simulink model "VentilatorClosedLoop_gas_f"  (R2018b)
settings: Solver=ode23t  StartTime=0.0  StopTime=50  MaxStep=0.001  RelTol=1e-3  EnableMultiTasking=on
PreLoadFcn:
  | loadVars
values from neighbouring files (symbols this model uses):
  basePSI = 14.7    [loadVars.m]
  D = 0.001    [loadVars.m]
  I = 0.2    [loadVars.m]
  P = 0.2    [loadVars.m]
libraries: fl_lib x26, nesl_utility x9, simulink x2, dspstat3 x1
(part 1 of 3)
settings Model: Creator=szhang  LastModifiedBy=etzorako
settings OptimizationCC: UseDivisionForNetSlopeComputation=on  LifeSpan=inf
settings DebuggingCC: LibraryContextMissingDiagnostic=none  SFUnexpectedBacktrackingDiag=warning  SFNoUnconditionalDefaultTransitionDiag=warning  SFExecutionAtInitializationDiag=none
settings SFSimCC: SimUseLocalCustomCode=off
settings RTWCC: RTWUseLocalCustomCode=off
settings CodeAppCC: StateflowObjectComments=on
settings GRTTargetCC: TargetLangStandard=C89/C90 (ANSI)  GeneratePreprocessorConditionals=Disable all
settings ConfigComp: CovMetricSettings=dw  CovHtmlReporting=on  CovSaveCumulativeToWorkspaceVar=on  CovSaveSingleToWorkspaceVar=on  CovExternalEMLEnable=off
settings SimscapeCC: SimscapeNormalizeSystem=off  SimscapeLogLimitData=off

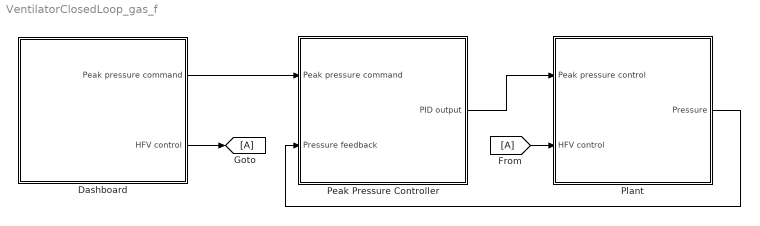
== system VentilatorClosedLoop_gas_f ==
  Dashboard : Subsystem
  Peak Pressure Controller : Subsystem
  Plant : Subsystem
  wires:
  [A] -> Plant/2(HFV control)
  Plant/1(Pressure) -> Peak Pressure Controller/2(Pressure feedback)
  Peak Pressure Controller/1(PID output) -> Plant/1(Peak pressure control)
  Dashboard/1(Peak pressure command) -> Peak Pressure Controller/1(Peak pressure command)
  Dashboard/2(HFV control) -> [A]

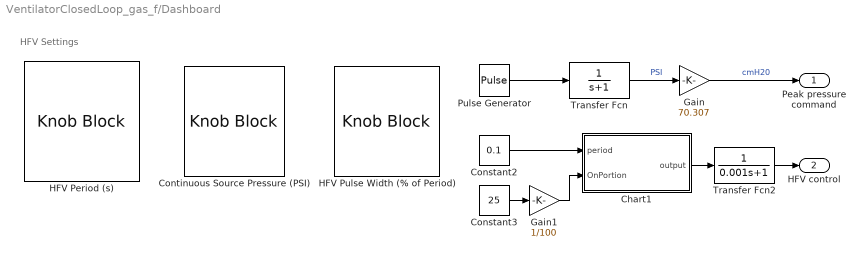
== system VentilatorClosedLoop_gas_f/Dashboard ==
  note: HFV Settings
  Chart1 : Stateflow chart  TreatAsAtomicUnit=on
  Constant2 : Constant  Value=0.1
  Constant3 : Constant  Value=25
  Continuous Source Pressure (PSI) : KnobBlock  WebBlockId=345  LabelPosition=Hide  ScaleMax=70  TickInterval=5
  Gain : Gain  Gain=70.307
  Gain1 : Gain  Gain=1/100
  HFV Period (s) : KnobBlock  WebBlockId=340  LabelPosition=Hide  ScaleMin=0.050000000000000003  ScaleMax=1  TickInterval=0.10000000000000001
  HFV Pulse Width (% of Period) : KnobBlock  WebBlockId=341  LabelPosition=Hide  ScaleMin=10  ScaleMax=50  TickInterval=5
  Pulse Generator : DiscretePulseGenerator  PulseType=Time based  Amplitude=0.3  Period=20  PulseWidth=50
  Transfer Fcn : TransferFcn  Denominator=[1 1]
  Transfer Fcn2 : TransferFcn  Denominator=[0.001 1]
  Peak pressure command : Outport
  HFV control : Outport  Port=2
  wires:
  Transfer Fcn/1 -> Gain/1  "PSI"
  Pulse Generator/1 -> Transfer Fcn/1
  Gain/1 -> Peak pressure command/1  "cmH20"
  Constant3/1 -> Gain1/1
  Chart1/1(output) -> Transfer Fcn2/1
  Constant2/1 -> Chart1/1(period)
  Gain1/1 -> Chart1/2(OnPortion)
  Transfer Fcn2/1 -> HFV control/1

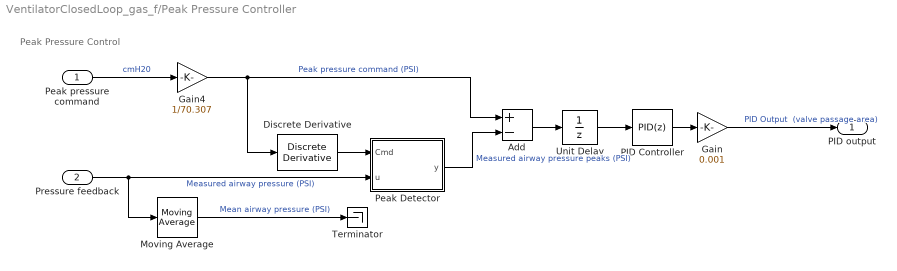
== system VentilatorClosedLoop_gas_f/Peak Pressure Controller ==
  note: Peak Pressure Control
  Peak pressure command : Inport  OutMin=0  OutMax=25  OutDataTypeStr=double  PortDimensions=1  SampleTime=0.001
  Pressure feedback : Inport  Port=2  OutMin=0  OutMax=1  OutDataTypeStr=double  PortDimensions=1  SampleTime=0.001
  Add : Sum  Inputs=+-
  Discrete Derivative : simulink/Discrete/Discrete Derivative  gainval=1.0  ICPrevScaledInput=0.0  OutMin=[]  OutMax=[]  OutDataType=fixdt(1, 16)  OutScaling=2^-10  DoSatur=off
  Gain : Gain  Gain=0.001
  Gain4 : Gain  Gain=1/70.307
  Moving Average : dspstat3/Moving Average  Method=Sliding window  ForgettingFactorPort=off  SpecifyWindowLength=on  WindowLength=200  ForgettingFactor=0.9  SimulateUsing=Code generation
  PID Controller : simulink/Continuous/PID Controller  Controller=PID  Form=Parallel  TimeDomain=Discrete-time  SampleTime=0.001  IntegratorMethod=Forward Euler  FilterMethod=Forward Euler  ControllerParametersSource=internal  P=P  I=I  D=D  UseFilter=on  N=100  TunerSelectOption=Transfer Function Based (PID Tuner App)  InitialConditionSource=internal  InitialConditionForIntegrator=0  InitialConditionForFilter=0  DifferentiatorICPrevScaledInput=0  ExternalReset=none  TrackingMode=off  Kt=1  LimitOutput=on  UpperSaturationLimit=0.5  LowerSaturationLimit=0  LinearizeAsGain=on  AntiWindupMode=clamping  Kb=1  POutMin=[]  POutMax=[]  IOutMin=[]  IOutMax=[]  DOutMin=[]  DOutMax=[]  NOutMin=[]  NOutMax=[]  SumOutMin=[]  SumOutMax=[]  SaturationOutMin=[]  SaturationOutMax=[]  PParamMin=[]  PParamMax=[]  IParamMin=[]  IParamMax=[]  DParamMin=[]  DParamMax=[]  NParamMin=[]  NParamMax=[]  KbParamMin=[]  KbParamMax=[]  KtParamMin=[]  KtParamMax=[]  KbOutMin=[]  KbOutMax=[]  KtOutMin=[]  KtOutMax=[]  IntegratorOutMin=[]  IntegratorOutMax=[]  FilterOutMin=[]  FilterOutMax=[]  SumI1OutMin=[]  SumI1OutMax=[]  SumI2OutMin=[]  SumI2OutMax=[]  SumI3OutMin=[]  SumI3OutMax=[]  SumI4OutMin=[]  SumI4OutMax=[]  SumDOutMin=[]  SumDOutMax=[]  DifferentiatorOutMin=[]  DifferentiatorOutMax=[]  FilterDiffOutCoefMin=[]  FilterDiffOutCoefMax=[]  ReciprocalOutMin=[]  ReciprocalOutMax=[]  SumDenOutMin=[]  SumDenOutMax=[]  SumNumOutMin=[]  SumNumOutMax=[]  DivideOutMin=[]  DivideOutMax=[]  IntegratorContinuousStateAttributes=''  IntegratorStateMustResolveToSignalObject=off  IntegratorRTWStateStorageClass=Auto  FilterContinuousStateAttributes=''  FilterStateMustResolveToSignalObject=off  FilterRTWStateStorageClass=Auto  ParallelPVariant=InternalParameters  IdealPVariant=Disabled  IVariant=InternalParameters  DVariant=InternalParameters  IntegratorVariant=Discrete  SatVariant=Enabled  AWVariant=DiscClampingParallel  PCopyVariant=Disabled  TRVariant=Disabled  FdbkBlocksVariant=Forward  IdealPFdbkVariant=Disabled  SatFdbkVariant=Disabled  DerivativeFilterVariant=ForwardEulerFilter  NVariant=InternalParameters  NCopyVariant=Disabled  FilterICVariant=InternalICsFilter  IntegratorICVariant=InternalICs  ExternalResetVariant=Disabled  TRSumVariant=Passthrough  SumFdbkVariant=Disabled  SumVariant=Sum_PID
  Peak Detector : MATLAB Function  TreatAsAtomicUnit=on
  Terminator : Terminator
  Unit Delay : UnitDelay  SampleTime=0.001
  PID output : Outport  OutMin=0  OutMax=1  OutDataTypeStr=double  PortDimensions=1  SampleTime=0.001
  wires:
  Gain4/1 -> Discrete Derivative/1, Add/1  "Peak pressure command (PSI)"
  Pressure feedback/1 -> Moving Average/1, Peak Detector/2(u)  "Measured airway pressure (PSI)"
  PID Controller/1 -> Gain/1
  Add/1 -> Unit Delay/1
  Unit Delay/1 -> PID Controller/1
  Gain/1 -> PID output/1  "PID Output  (valve passage area)"
  Peak pressure command/1 -> Gain4/1  "cmH20"
  Peak Detector/1(y) -> Add/2  "Measured airway pressure peaks (PSI)"
  Discrete Derivative/1 -> Peak Detector/1(Cmd)
  Moving Average/1 -> Terminator/1  "Mean airway pressure (PSI)"
